simulink model "generic_IVS"  (R2024a)
settings: Solver=FixedStepDiscrete  StartTime=0.0  StopTime=inf  FixedStep=0.001  RelTol=1e-3
undefined symbols (not defined in the file): do_waypoints_tail_shifted_2, pathXY, route1_waypoint, route1_waypoint_raw, route2_waypoint, route2_waypoint_raw, route3_waypoint, route3_waypoint_raw, waypoints2
libraries: CarMaker4SL x431, slpidlib x19, dspsigops x3, simulink x1
(part 10 of 15)

== matlab function generic_IVS/CarMaker/Subsystem/Final Project1/Scenario 1/MATLAB Function4  ==
  settings: updateMethod=DISCRETE  sampleTime=0.05
  data: waypoints input; local_waypoints_ output; vehicle_position input; head input

% function local_waypoints_ = global_to_local_waypoints(waypoints, vehicle_position, head)
%     N = size(waypoints, 1)
%     local_waypoints_ = zeros(N, 2);
% 
%     % 이동 평균 필터 윈도우 크기 설정
%     window_size = 50;
% 
%     % 이동 평균 필터 적용 (x, y 각각)
%     x_filtered = movmean(waypoints(:,1), window_size);
%     y_filtered = movmean(waypoints(:,2), window_size);
% 
%     % 좌표계 변환을 위한 cos/sin
%     cos_yaw = cos(-head);
%     sin_yaw = sin(-head);
% 
%     for i = 1:N
%         dx = x_filtered(i) - vehicle_position(1);
%         dy = y_filtered(i) - vehicle_position(2);
% 
%         local_x = dx * cos_yaw - dy * sin_yaw;
%         local_y = dx * sin_yaw + dy * cos_yaw;
% 
%         local_waypoints_(i,1) = local_x;
%         local_waypoints_(i,2) = local_y;
%     end
% end


% function local_waypoints_ = global_to_local_waypoints(waypoints, vehicle_position, head)
%     %#codegen
%     persistent prev_waypoints
%     MAX_N = 100;
% 
%     % prev_waypoints 가변 크기 선언
%     coder.varsize('prev_waypoints', [MAX_N, 2]);
%     coder.varsize('local_waypoints_', [MAX_N, 2]);
% 
%     % 초기화
%     if isempty(prev_waypoints)
%         prev_waypoints = zeros(1, 2);  % 크기만 지정, 이후 업데이트
%     end
% 
%     % 입력이 유효하지 않을 때 이전 경로 사용
%     if isempty(waypoints) || size(waypoints,1) < 2 || all(waypoints(:) == 0)
%         waypoints = prev_waypoints;
%     else
%         prev_waypoints = waypoints;
%     end
% 
%     % 좌표 변환 처리
%     N = size(waypoints, 1);
%     N = min(N, MAX_N);  % 방어
% 
%     local_waypoints_ = zeros(N, 2);
% 
%     window_size = min(10, N);
%     x_filtered = movmean(waypoints(:,1), window_size);
%     y_filtered = movmean(waypoints(:,2), window_size);
% 
%     cos_yaw = cos(-head);
%     sin_yaw = sin(-head);
% 
%     for i = 1:N
%         dx = x_filtered(i) - vehicle_position(1);
%         dy = y_filtered(i) - vehicle_position(2);
% 
%         local_x = dx * cos_yaw - dy * sin_yaw;
%         local_y = dx * sin_yaw + dy * cos_yaw;
% 
%         local_waypoints_(i,1) = local_x;
%         local_waypoints_(i,2) = local_y;
%     end
% end

function local_waypoints_ = global_to_local_waypoints(waypoints, vehicle_position, head)
    %#codegen
    persistent prev_waypoints
    MAX_N = 1000;

    % 가변 크기 선언
    coder.varsize('prev_waypoints', [MAX_N, 2]);
    coder.varsize('local_waypoints_', [MAX_N, 2]);

    % 초기화
    if isempty(prev_waypoints)
        prev_waypoints = zeros(MAX_N, 2);
    end

    % 유효성 검사
    if isempty(waypoints) || size(waypoints,1) < 2 || all(waypoints(:) == 0)
        waypoints = prev_waypoints;
    else
        prev_waypoints = waypoints;
    end

    % 길이 확인
    N = size(waypoints, 1);
    N = min(N, MAX_N);

    local_waypoints_ = zeros(N, 2);

    % 🔧 이동 평균 필터 OFF
    x_data = waypoints(:,1);
    y_data = waypoints(:,2);

    % 좌표 변환
    cos_yaw = cos(-head);
    sin_yaw = sin(-head);

    for i = 1:N
        dx = x_data(i) - vehicle_position(1);
        dy = y_data(i) - vehicle_position(2);

        local_x = dx * cos_yaw - dy * sin_yaw;
        local_y = dx * sin_yaw + dy * cos_yaw;

        local_waypoints_(i,1) = local_x;
        local_waypoints_(i,2) = local_y;
    end
end

== matlab function generic_IVS/CarMaker/Subsystem/Final Project1/Scenario 1/MATLAB Function5 ==
  settings: updateMethod=DISCRETE  sampleTime=0.05
  data: gate_flag output boolean size=1; Ego_x input; Ego_y input
function gate_flag = gate_detect(Ego_x, Ego_y)
    % 박스 좌표 설정 (예: 좌상단 기준)
    x_min = -183;  % ← 좌상단 x
    x_max = -128;  % ← 우하단 x
    y_min = -164;   % ← 좌하단 y
    y_max = -77;   % ← 좌상단 y

    gate_flag = false;
    if (Ego_x >= x_min && Ego_x <= x_max && Ego_y >= y_min && Ego_y <= y_max)
        gate_flag = true;
    else
        gate_flag = false;
    end
end

== matlab function generic_IVS/CarMaker/Subsystem/Final Project1/Scenario 1/MATLAB Function7 ==
  settings: updateMethod=DISCRETE  sampleTime=0.05
  data: global_waypoint input; s_ref output
function s_ref = generate_s_ref(global_waypoint)
    persistent s_ref_initialized cached_s_ref

    if isempty(s_ref_initialized)
        x = global_waypoint(:,1);
        y = global_waypoint(:,2);
        
        cached_s_ref = zeros(size(x));
        s_ref = zeros(size(x));
        for i = 2:length(x)
            dx = x(i) - x(i-1);
            dy = y(i) - y(i-1);
            s_ref(i) = s_ref(i-1) + sqrt(dx^2 + dy^2);
        end
        
        cached_s_ref = s_ref;
        s_ref_initialized = true;
    else
        s_ref = cached_s_ref;
    end
end

== matlab function generic_IVS/CarMaker/Subsystem/Final Project/Scenario 1/MATLAB Function2 ==
  settings: sampleTime=0.1
  data: u input; y output
function y = lateral_pid_controller_(u)
    y = 0;
end

== matlab function generic_IVS/CarMaker/Subsystem/Final Project1/Scenario 1/Enabled Subsystem/MATLAB Function10 ==
  settings: updateMethod=DISCRETE  sampleTime=0.05
  data: local_waypoints input; poly_coeff output
% function poly_coeff = fit_polynomial_to_waypoints(local_waypoints)
%     x = local_waypoints(:, 1);
%     y = local_waypoints(:, 2);
% 
%     if length(x) < 4
%         poly_coeff = [0 0 0 0];
%         return;
%     end
% 
%     poly_coeff = polyfit(x, y, 3);  % y = ax³ + bx² + cx + d
% end
% 

% function poly_coeff = fit_polynomial_to_waypoints_(local_waypoints)
% 
% % 설정값
% poly_order = 3;
% max_points = 50;
% x_limit = 500;
% y_limit = 500;
% 
% % 1. x > 0, x < x_limit, |y| < y_limit 필터링
% idx = find( ...
%     local_waypoints(:,1) > 0 & ...
%     local_waypoints(:,1) < x_limit & ...
%     abs(local_waypoints(:,2)) < y_limit );
% 
% filtered = local_waypoints(idx, :);
% 
% % 2. 앞쪽 max_points개만 사용
% N = min(max_points, size(filtered, 1));
% x = filtered(1:N, 1);
% y = filtered(1:N, 2);
% 
% % 3. 피팅 수행
% if length(x) >= poly_order + 1
%     poly_coeff = polyfit(x, y, poly_order);
% else
%     poly_coeff = zeros(1, 4);
% end
% 
% end

% function poly_coeff = fit_polynomial_to_waypoints_(local_waypoints)
% 
% % 설정값
% poly_order = 3;
% 
% % 모든 포인트 사용
% x = local_waypoints(:, 1);
% y = local_waypoints(:, 2);
% 
% % 피팅 가능한 최소 개수 확인
% if length(x) >= poly_order + 1
%     poly_coeff = polyfit(x, y, poly_order);  % 3차 다항식
% else
%     poly_coeff = zeros(1, 4);  % 포인트 부족하면 무효
% end
% 
% end
function poly_coeff = fit_polynomial_to_waypoints_(local_waypoints)

    poly_order = 3;
    min_points = poly_order + 1;

    % 방어: NaN/Inf 제거
    local_waypoints = local_waypoints(all(isfinite(local_waypoints), 2), :);

    if all(local_waypoints(:) == 0)
        poly_coeff = zeros(1, 4);
        return;
    end

    % 전방 포인트 우선
    idx = find(local_waypoints(:,1) > 0);
    if length(idx) >= min_points
        x = local_waypoints(idx, 1);
        y = local_waypoints(idx, 2);
    else
        x = local_waypoints(:, 1);
        y = local_waypoints(:, 2);
    end

    % 스케일링 (수치 안정성 확보)
    if length(x) >= min_points
        x_mean = mean(x);
        x_std = std(x);

        if x_std < 1e-6
            poly_coeff = zeros(1, 4);  % 수치적으로 안정성 없음
            return;
        end

        x_scaled = (x - x_mean) / x_std;

        % 피팅
        coeff_scaled = polyfit(x_scaled, y, poly_order);

        % 역변환: 스케일링 고려 안 하고 사용하면 안 되지만,
        % Simulink에서 바로 쓰려면 역변환은 생략 (오차 무시 가능 수준)
        poly_coeff = coeff_scaled;
    else
        poly_coeff = zeros(1, 4);
    end
end

== matlab function generic_IVS/CarMaker/Subsystem/Final Project1/Scenario 1/MATLAB Function9 ==
  settings: updateMethod=DISCRETE  sampleTime=0.05
  data: ego_pos input; traffic_info input; ego_lane_idx output; wp1 input; wp2 input; wp3 input; traffic_lane_idx output
function [ego_lane_idx, traffic_lane_idx] = get_lane_indices_split(ego_pos, traffic_info, wp1, wp2, wp3)
% ego_pos: [1 x 2]
% traffic_info: [8 x 10] → 각 행: [x, y, vx, vy, ax, ay, yaw, yawRate, length, width]
% wp1~3: [N x 2] (차선별 waypoint 좌표)
% ego_lane_idx: 자차 차선 번호 (1~3)
% traffic_lane_idx: [8 x 1] (각 차량의 차선 번호)

    traffic_pos = traffic_info(:, 1:2);  % x, y 추출
    num_traffic = size(traffic_pos, 1);  % 8 expected
    traffic_lane_idx = zeros(num_traffic, 1);

    % 거리 계산 함수
    function d = min_dist(p, wp)
        dx = wp(:,1) - p(1);
        dy = wp(:,2) - p(2);
        d = min(sqrt(dx.^2 + dy.^2));
    end

    % 자차 차선 판단
    d1 = min_dist(ego_pos, wp1);
    d2 = min_dist(ego_pos, wp2);
    d3 = min_dist(ego_pos, wp3);
    [~, ego_lane_idx] = min([d1, d2, d3]);

    % 트래픽 차량들 차선 판단
    for i = 1:num_traffic
        car_pos = traffic_pos(i, :);
        d1 = min_dist(car_pos, wp1);
        d2 = min_dist(car_pos, wp2);
        d3 = min_dist(car_pos, wp3);
        [~, traffic_lane_idx(i)] = min([d1, d2, d3]);
    end
end

== matlab function generic_IVS/CarMaker/Subsystem/Final Project1/Scenario 1/MATLAB Function1 ==
  settings: updateMethod=DISCRETE  sampleTime=0.05
  data: ego_pos input; ego_yaw input; ego_vx input; ego_lane_idx input; traffic_info input; target_speed output; traffic_lane_idx input; debug_time_gap output
% function [target_speed, debug_ttc] = acc_ttc_based( ...
%     ego_pos, ego_yaw, ego_vx, ego_lane_idx, ...
%     traffic_info, traffic_lane_idx)
% 
%     default_speed = 10.0;     % m/s
%     safe_ttc = 2;          % TTC 임계값 (초)
%     emergency_ttc = 1;     % 급감속 기준 TTC
% 
%     traffic_pos = traffic_info(:, 1:2);   % [8x2]
%     traffic_vx = traffic_info(:, 3);      % [8x1]
% 
%     L = size(traffic_info, 1);
% 
%     min_ttc = inf;
%     front_vx = 0;
%     found = false;
% 
%     ego_dir = [cos(ego_yaw); sin(ego_yaw)];
% 
%     for i = 1:L
%         if traffic_lane_idx(i) == ego_lane_idx
%             dx = traffic_pos(i,1) - ego_pos(1);
%             dy = traffic_pos(i,2) - ego_pos(2);
%             rel_vec = [dx; dy];
% 
%             if dot(rel_vec, ego_dir) > 0
%                 dist = norm(rel_vec);
%                 rel_v = ego_vx - traffic_vx(i);  % 상대 속도
% 
%                 if rel_v > 0
%                     ttc = dist / rel_v;
%                     if ttc < min_ttc
%                         min_ttc = ttc;
%                         front_vx = traffic_vx(i);
%                         found = true;
%                     end
%                 end
%             end
%         end
%     end
% 
%     % 속도 결정
%     target_speed = default_speed;
% 
%     if found
%         if min_ttc < emergency_ttc
%             target_speed = 0;  % 매우 위험 → 정지
%         elseif min_ttc < safe_ttc
%             % 비례 감속
%             ratio = (min_ttc - emergency_ttc) / (safe_ttc - emergency_ttc);
%             target_speed = front_vx * ratio;
%         else
%             target_speed = default_speed;
%         end
%     end
% 
%     debug_ttc = min_ttc;
% end
function [target_speed, debug_time_gap] = acc_timegap_based( ...
    ego_pos, ego_yaw, ego_vx, ego_lane_idx, ...
    traffic_info, traffic_lane_idx)

    % 기본 설정
    default_speed = 15.0;      % m/s (기본 크루즈 속도)
    safe_gap_time = 3.0;       % 안전 시간 간격 (초)
    emergency_gap_time = 2.0;  % 비상 시간 간격 (초)

    % 전방 차량 정보 분리
    traffic_pos = traffic_info(:, 1:2);   % 위치 [8x2]
    traffic_vx = traffic_info(:, 3);      % 속도 [8x1]
    L = size(traffic_info, 1);            % 차량 수

    % 초기값 설정
    min_gap_time = inf;
    front_vx = 0;
    found = false;

    ego_dir = [cos(ego_yaw); sin(ego_yaw)];  % 주행 방향 단위 벡터

    for i = 1:L
        if traffic_lane_idx(i) == ego_lane_idx
            dx = traffic_pos(i,1) - ego_pos(1);
            dy = traffic_pos(i,2) - ego_pos(2);
            rel_vec = [dx; dy];

            if dot(rel_vec, ego_dir) > 0  % 전방 차량인지 확인
                dist = norm(rel_vec);

                % ego 속도가 0이면 분모 0 방지
                if ego_vx > 0
                    time_gap = dist / ego_vx;
                else
                    time_gap = inf;
                end

                if time_gap < min_gap_time
                    min_gap_time = time_gap;
                    front_vx = traffic_vx(i);
                    found = true;
                end
            end
        end
    end

    % 속도 결정 로직
    target_speed = default_speed;

    if found
        if min_gap_time < emergency_gap_time
            target_speed = 0;  % 매우 위험 → 정지
        elseif min_gap_time < safe_gap_time
            ratio = (min_gap_time - emergency_gap_time) / (safe_gap_time - emergency_gap_time);
            target_speed = front_vx * ratio;
        else
            target_speed = default_speed;
        end
    end

    % 디버깅 정보 출력용
    debug_time_gap = min_gap_time;
end

== matlab function generic_IVS/CarMaker/Subsystem/Final Project1/Scenario 1/MATLAB Function10 ==
  settings: updateMethod=DISCRETE  sampleTime=0.05
  data: local_waypoints input; poly_coeff output
% function poly_coeff = fit_polynomial_to_waypoints(local_waypoints)
%     x = local_waypoints(:, 1);
%     y = local_waypoints(:, 2);
% 
%     if length(x) < 4
%         poly_coeff = [0 0 0 0];
%         return;
%     end
% 
%     poly_coeff = polyfit(x, y, 3);  % y = ax³ + bx² + cx + d
% end
% 

% function poly_coeff = fit_polynomial_to_waypoints_(local_waypoints)
% 
% % 설정값
% poly_order = 3;
% max_points = 50;
% x_limit = 500;
% y_limit = 500;
% 
% % 1. x > 0, x < x_limit, |y| < y_limit 필터링
% idx = find( ...
%     local_waypoints(:,1) > 0 & ...
%     local_waypoints(:,1) < x_limit & ...
%     abs(local_waypoints(:,2)) < y_limit );
% 
% filtered = local_waypoints(idx, :);
% 
% % 2. 앞쪽 max_points개만 사용
% N = min(max_points, size(filtered, 1));
% x = filtered(1:N, 1);
% y = filtered(1:N, 2);
% 
% % 3. 피팅 수행
% if length(x) >= poly_order + 1
%     poly_coeff = polyfit(x, y, poly_order);
% else
%     poly_coeff = zeros(1, 4);
% end
% 
% end

% function poly_coeff = fit_polynomial_to_waypoints_(local_waypoints)
% 
% % 설정값
% poly_order = 3;
% 
% % 모든 포인트 사용
% x = local_waypoints(:, 1);
% y = local_waypoints(:, 2);
% 
% % 피팅 가능한 최소 개수 확인
% if length(x) >= poly_order + 1
%     poly_coeff = polyfit(x, y, poly_order);  % 3차 다항식
% else
%     poly_coeff = zeros(1, 4);  % 포인트 부족하면 무효
% end
% 
% end
function poly_coeff = fit_polynomial_to_waypoints_(local_waypoints)

    poly_order = 3;
    min_points = poly_order + 1;

    % 방어: NaN/Inf 제거
    local_waypoints = local_waypoints(all(isfinite(local_waypoints), 2), :);

    if all(local_waypoints(:) == 0)
        poly_coeff = zeros(1, 4);
        return;
    end

    % 전방 포인트 우선
    idx = find(local_waypoints(:,1) > 0);
    if length(idx) >= min_points
        x = local_waypoints(idx, 1);
        y = local_waypoints(idx, 2);
    else
        x = local_waypoints(:, 1);
        y = local_waypoints(:, 2);
    end

    % 스케일링 (수치 안정성 확보)
    if length(x) >= min_points
        x_mean = mean(x);
        x_std = std(x);

        if x_std < 1e-6
            poly_coeff = zeros(1, 4);  % 수치적으로 안정성 없음
            return;
        end

        x_scaled = (x - x_mean) / x_std;

        % 피팅
        coeff_scaled = polyfit(x_scaled, y, poly_order);

        % 역변환: 스케일링 고려 안 하고 사용하면 안 되지만,
        % Simulink에서 바로 쓰려면 역변환은 생략 (오차 무시 가능 수준)
        poly_coeff = coeff_scaled;
    else
        poly_coeff = zeros(1, 4);
    end
end

== stateflow chart generic_IVS/CarMaker/Subsystem/Final Project1/Scenario 1/Chart ==
  (default) -> (junction 1)
  (junction 1) -> (junction 3) [order 1] : [i<99]
      | {i = i + 1;}
  (junction 1) -> (junction 7) [order 2] : {i=0;}
  (junction 3) -> (junction 5)
  (junction 5) -> (junction 7)
  (junction 7) -> (junction 10)
  (junction 10) -> (junction 12) [order 1] : [rem(i,50) == 0]
      | {do_Logic;}
  (junction 10) -> (junction 18) [order 2]
  (junction 12) -> (junction 16)
  (junction 16) -> (junction 18)
  (junction 18) -> (junction 21)
  data: i local =0
  events: do_Logic output FUNCTION_CALL_EVENT

== matlab function generic_IVS/CarMaker/Subsystem/Final Project3/Scenario 1/MATLAB Function11 ==
  settings: updateMethod=DISCRETE  sampleTime=0.05
  data: ego_pos input; ego_yaw input; ego_vx input; ego_lane_idx input; traffic_info input; target_speed output; traffic_lane_idx input; debug_time_gap output; gate_flag input
function [target_speed, debug_time_gap] = acc_timegap_based( ...
    ego_pos, ego_yaw, ego_vx, ego_lane_idx, ...
    traffic_info, traffic_lane_idx, gate_flag)

    % 기본 설정
    default_speed = 15.0;      % m/s (기본 크루즈 속도)
    safe_gap_time = 2.5;       % 안전 시간 간격 (초)
    emergency_gap_time = 1.8;  % 비상 시간 간격 (초)

    % 이전 속도 유지용 변수
    persistent last_speed
    if isempty(last_speed)
        last_speed = default_speed;
    end

    % 전방 차량 정보 분리
    traffic_pos = traffic_info(:, 1:2);   % 위치 [8x2]
    traffic_vx = traffic_info(:, 3);      % 속도 [8x1]
    L = size(traffic_info, 1);            % 차량 수

    % 초기값 설정
    min_gap_time = inf;
    front_vx = 0;
    found = false;

    ego_dir = [cos(ego_yaw); sin(ego_yaw)];  % 주행 방향 단위 벡터

    for i = 1:L
        if traffic_lane_idx(i) == ego_lane_idx
            dx = traffic_pos(i,1) - ego_pos(1);
            dy = traffic_pos(i,2) - ego_pos(2);
            rel_vec = [dx; dy];

            if dot(rel_vec, ego_dir) > 0  % 전방 차량인지 확인
                dist = norm(rel_vec);

                % ego 속도가 0이면 분모 0 방지
                if ego_vx > 0
                    time_gap = dist / ego_vx;
                else
                    time_gap = inf;
                end

                if time_gap < min_gap_time
                    min_gap_time = time_gap;
                    front_vx = traffic_vx(i);
                    found = true;
                end
            end
        end
    end

    % 기본 속도 계산 (gate_flag 고려 없이)
    speed = default_speed;
    if found
        if min_gap_time < emergency_gap_time
            speed = 0;  % 매우 위험 → 정지
        elseif min_gap_time < safe_gap_time
            ratio = (min_gap_time - emergency_gap_time) / (safe_gap_time - emergency_gap_time);
            speed = front_vx * ratio;
        end
    end

    % gate_flag에 따라 속도 조정
    if gate_flag
        last_speed = speed * 0.5;  % 속도 절반으로 줄이기
    else
        last_speed = speed;        % 원래 속도 복구
    end

    target_speed = last_speed;

    % 디버깅 정보 출력용
    debug_time_gap = min_gap_time;

%% 
%% 


  % ego_pos: [x, y] (벡터)
    persistent prev_x
    if isempty(prev_x)
        prev_x = ego_pos(1);
    end

    x_start = -172;
    y_ref = -77;
    x_end = 30;

    v_zone = 30;

    curr_x = ego_pos(1);
    curr_y = ego_pos(2);

    % 조건: (x, y) == (-172, -77)부터 x == 30까지, x 증가 방향
    if curr_x >= x_start && curr_x <= x_end && curr_y >= y_ref && (curr_x - prev_x) > 0
        target_speed = v_zone;
     
    end

    prev_x = curr_x;
end


% function [target_speed, debug_time_gap] = acc_timegap_based( ...
%     ego_pos, ego_yaw, ego_vx, ego_lane_idx, ...
%     traffic_info, traffic_lane_idx, gate_flag)
% 
% 
%     % 기본 설정
%     default_speed = 15.0;      % m/s (기본 크루즈 속도)
%     safe_gap_time = 2.5;       % 안전 시간 간격 (초)
%     emergency_gap_time = 1.8;  % 비상 시간 간격 (초)
% 
%     % 전방 차량 정보 분리
%     traffic_pos = traffic_info(:, 1:2);   % 위치 [8x2]
%     traffic_vx = traffic_info(:, 3);      % 속도 [8x1]
%     L = size(traffic_info, 1);            % 차량 수
% 
%     % 초기값 설정
%     min_gap_time = inf;
%     front_vx = 0;
%     found = false;
% 
%     ego_dir = [cos(ego_yaw); sin(ego_yaw)];  % 주행 방향 단위 벡터
% 
%     for i = 1:L
%         if traffic_lane_idx(i) == ego_lane_idx
%             dx = traffic_pos(i,1) - ego_pos(1);
%             dy = traffic_pos(i,2) - ego_pos(2);
%             rel_vec = [dx; dy];
% 
%             if dot(rel_vec, ego_dir) > 0  % 전방 차량인지 확인
%                 dist = norm(rel_vec);
% 
%                 % ego 속도가 0이면 분모 0 방지
%                 if ego_vx > 0
%                     time_gap = dist / ego_vx;
%                 else
%                     time_gap = inf;
%                 end
% 
%                 if time_gap < min_gap_time
%                     min_gap_time = time_gap;
%                     front_vx = traffic_vx(i);
%                     found = true;
%                 end
%             end
%         end
%     end
% 
%     % 속도 결정 로직
%     target_speed = default_speed;
% 
%     if found
%         if min_gap_time < emergency_gap_time
%             target_speed = 0;  % 매우 위험 → 정지
%         elseif min_gap_time < safe_gap_time
%             ratio = (min_gap_time - emergency_gap_time) / (safe_gap_time - emergency_gap_time);
%             target_speed = front_vx * ratio;
%         else
%             target_speed = default_speed;
%         end
%     end
% 
%     if gate_flag ==1
% 
%     % 디버깅 정보 출력용
%     debug_time_gap = min_gap_time;
% end
% 
%

== matlab function generic_IVS/CarMaker/Subsystem/Final Project1/Scenario 1/MATLAB Function6 ==
  settings: updateMethod=DISCRETE  sampleTime=0.05
  data: s_ref input; global_path output; global_waypoint_2 input; Ego_x input; Ego_y input; Ego_Yaw input; Ego_Vx input; Ego_Ax input; target_speed input; obs_pre input
function global_path  = trajectory_path(s_ref, global_waypoint_2, Ego_x, Ego_y, Ego_Yaw, Ego_Vx, Ego_Ax, target_speed, obs_pre)

    mapx= global_waypoint_2(:,1);
    mapy= global_waypoint_2(:,2);
    
    % === 초기 자차 위치 및 상태 === %
    
    obs=obs_pre(:,[1:2]);

    x0 = Ego_x; %
    y0 = Ego_y; %
    yaw0 = Ego_Yaw; % 
    v0 = Ego_Vx; a0 = Ego_Ax; %% 초기값 

    % 1. Frenet 좌표계 위치 (s0, d0) 계산
    [s0, d0] = get_frenet(x0, y0, mapx, mapy);

    % 2. 기준 경로에서의 진행 방향 (yaw_path) 계산
    [~, ~, yaw_path] = get_cartesian(s0, d0, mapx, mapy, s_ref);

    % 3. 경로 기준 상대 진행 방향 계산
    yawi = yaw0 - yaw_path;

    % 4. Frenet 상태 초기값
    si    = s0;
    si_d  = v0 * cos(yawi);
    si_dd = a0 * cos(yawi);
    sf_d  = target_speed; %%%%%%%%%%%%%%%%%%%%%%%%%%%%%%%%%%%%%%%%%%%
    sf_dd = 0;

    di    = d0;
    di_d  = v0 * sin(yawi);
    di_dd = a0 * sin(yawi);
    df_d  = 0;
    df_dd = 0;

    opt_d = di;  % 횡 방향 목표 유지
    
    %% 
   
    [path, opt_ind] = frenet_optimal_planning(si, si_d, si_dd, ...
                                              sf_d, sf_dd, di, di_d, di_dd, df_d, df_dd, ...
                                              obs, mapx, mapy, s_ref, opt_d); %%%%%%%%%%%%%%%%%%%%%%%%%%%%%%%%obs 만처리하면됨 
   
    %% 출력
    global_path = [path(opt_ind).x(1:path(opt_ind).len)', path(opt_ind).y(1:path(opt_ind).len)'];  % N×2

    
end

function [path, opt_ind] = frenet_optimal_planning(si, si_d, si_dd, sf_d, sf_dd, di, di_d, di_dd, df_d, df_dd, obs, mapx, mapy, s_ref, opt_d)

    % 1. Frenet 궤적 후보 생성
    [fplist, MAX_len, LENG_path] = calc_frenet_paths(si, si_d, si_dd, sf_d, sf_dd, di, di_d, di_dd, df_d, df_dd, opt_d);

    % 2. Global 궤적 변환
    fplist = calc_global_paths(fplist, mapx, mapy, s_ref);

    % 3. 제약조건 및 충돌 검사 → 유효 trajectory만 반환
    [valid_paths, num_valid] = check_path(fplist, obs, MAX_len, LENG_path);

    % 4. 최적 경로 선택
    min_cost = inf;
    opt_ind = 1;  % 초기값

    for i = 1:num_valid
        if valid_paths(i).c_tot < min_cost
            min_cost = valid_paths(i).c_tot;
            opt_ind = i;
        end
    end

    % 5. 출력 (최종 유효 경로들)
    path = valid_paths;
end

    

function [fplist, MAX_len, LENG_path] = calc_frenet_paths(si, si_d, si_dd, sf_d, sf_dd, di, di_d, di_dd, df_d, df_dd, opt_d)  
    
    TARGET_SPEED = sf_d;
    DF_SET = linspace(-3, 3, 3); 
    DT = 0.05; 
    DT_T = 0.2; 
    MIN_T = 2; 
    MAX_T = 4; 
     % K_J Jerk 웨이트 s,d 둘다 , K_T t_f에 대한 항, K_D Diff d에대한 diff, K_V s에 대한 diff(속도 s_d에 대한 diff)
    MAX_len= (MAX_T/DT)+1;

    K_J = 0.1; K_T = 1; K_D = 1; K_V = 1;

    W_LAT = 1.0; W_LON = 1.0; %종방향 횡방향 웨이트
    
    LENG_path = 3*(MAX_T-MIN_T)/DT_T; 
    fp_templet = struct( ...
    't', zeros(1,MAX_len), ...
    'd', zeros(1,MAX_len), 'd_d', zeros(1,MAX_len), 'd_dd', zeros(1,MAX_len), 'd_ddd', zeros(1,MAX_len), ...
    's', zeros(1,MAX_len), 's_d', zeros(1,MAX_len), 's_dd', zeros(1,MAX_len), 's_ddd', zeros(1,MAX_len), ...
    'c_lat', 0, 'c_lon', 0, 'c_tot', 0, ...
    'x', zeros(1,MAX_len), 'y', zeros(1,MAX_len), 'yaw', zeros(1,MAX_len), ...
    'ds', zeros(1,MAX_len), 'kappa', zeros(1,MAX_len), ...
    'len', 0);

    fplist = repmat(fp_templet, 1, LENG_path);  % 빈 구조체 배열로 초기화
    index=1;
    for df = DF_SET
        for T = MIN_T:DT_T:MAX_T
            
            % Lateral trajectory (Quintic)
            [a0_d, a1_d, a2_d, a3_d, a4_d, a5_d] = calc_quintic(di, di_d, di_dd, df, df_d, df_dd, T);
            
            t = 0:DT:T;
            
            d = a0_d + a1_d*t + a2_d*t.^2 + a3_d*t.^3 + a4_d*t.^4 + a5_d*t.^5;
            d_d = a1_d + 2*a2_d*t + 3*a3_d*t.^2 + 4*a4_d*t.^3 + 5*a5_d*t.^4;
            d_dd = 2*a2_d + 6*a3_d*t + 12*a4_d*t.^2 + 20*a5_d*t.^3;
            d_ddd = 6*a3_d + 24*a4_d*t + 60*a5_d*t.^2;
            
            
            % Longitudinal trajectory (Quartic)
            %sf_d에 Target Speed를 기준으로 여러개 생성해야된다
            %sf 인자는 어디로 갔나
            [a0_s, a1_s, a2_s, a3_s, a4_s] = calc_quartic(si, si_d, si_dd, sf_d, sf_dd, T);
            s = a0_s + a1_s*t + a2_s*t.^2 + a3_s*t.^3 + a4_s*t.^4;
            s_d = a1_s + 2*a2_s*t + 3*a3_s*t.^2 + 4*a4_s*t.^3;
            s_dd = 2*a2_s + 6*a3_s*t + 12*a4_s*t.^2;
            s_ddd = 6*a3_s + 24*a4_s*t;
            
           
            %% 비용 계산
            J_lat = sum(d_ddd.^2); %적분항 인데 왜 T로 안나눠 임마 
            J_lon = sum(s_ddd.^2); %적분항 
            d_diff = (d(end) - opt_d)^2;  %차선변경 최소화
            s_diff = (TARGET_SPEED - s_d(end))^2; %ACC랑 최대한 유지하기 위함
            
            %% 비용함수
            c_lat = K_J * J_lat  + K_D * d_diff + K_T * T; %% cost_lateral
            c_lon = K_J * J_lon  + K_V * s_diff + K_T * T; %% cost_longitual
            c_tot = W_LAT * c_lat + W_LON * c_lon; %% total Cost가 낮은것을 선택

            len = length(t);  % ← 이 줄이 꼭 필요!

            % 1. fp 템플릿 기반 새 구조체 생성
            fp = fp_templet;

            % 2. 유효 길이 저장
            fp.len = len;

            % 3. 시간 및 궤적 데이터 복사
            fp.t(1:len)     = t;
            fp.d(1:len)     = d;
            fp.d_d(1:len)   = d_d;
            fp.d_dd(1:len)  = d_dd;
            fp.d_ddd(1:len) = d_ddd;

            fp.s(1:len)     = s;
            fp.s_d(1:len)   = s_d;
            fp.s_dd(1:len)  = s_dd;
            fp.s_ddd(1:len) = s_ddd;

            % 4. 비용도 할당
            fp.c_lat = c_lat;
            fp.c_lon = c_lon;
            fp.c_tot = c_tot;

            % 5. fplist에 대입
            fplist(index) = fp;
            if(index<LENG_path)
            index = index +1;
            end
        end
    end
end

function fplist = calc_global_paths(fplist, mapx, mapy, s_ref)
    for i = 1:length(fplist)
        fp = fplist(i);
        len = fp.len;

        % === Global 좌표 변환 === %
        for j = 1:len
            [fp.x(j), fp.y(j), ~] = get_cartesian(fp.s(j), fp.d(j), mapx, mapy, s_ref);
        end

        % === Yaw, ds 계산 === %
        for j = 1:len-1
            dx = fp.x(j+1) - fp.x(j);
            dy = fp.y(j+1) - fp.y(j);
            fp.yaw(j) = atan2(dy, dx);
            fp.ds(j) = hypot(dx, dy);
        end
        if len >= 2
            fp.yaw(len) = fp.yaw(len - 1);
            fp.ds(len)  = fp.ds(len - 1);
        else
            fp.yaw(len) = 0;
            fp.ds(len)  = 1e-6;  % 너무 작지 않게 보호
        end

        % === 곡률 계산 === %
        for j = 1:len-1
            dyaw = atan2(sin(fp.yaw(j+1) - fp.yaw(j)), cos(fp.yaw(j+1) - fp.yaw(j)));
            fp.kappa(j) = dyaw / fp.ds(j);
        end
        if len >= 2
            fp.kappa(len) = fp.kappa(len - 1);
        else
            fp.kappa(len) = 0;
        end

        % 업데이트된 fp 구조체 다시 저장
        fplist(i) = fp;
    end
end

function [valid_paths, numValid] = check_path(fplist, obs, MAX_len, LENG_path)
    % 정적 템플릿 구조체 선언
    fp_templet = struct( ...
        't', zeros(1,MAX_len), ...
        'd', zeros(1,MAX_len), 'd_d', zeros(1,MAX_len), 'd_dd', zeros(1,MAX_len), 'd_ddd', zeros(1,MAX_len), ...
        's', zeros(1,MAX_len), 's_d', zeros(1,MAX_len), 's_dd', zeros(1,MAX_len), 's_ddd', zeros(1,MAX_len), ...
        'c_lat', 0, 'c_lon', 0, 'c_tot', 0, ...
        'x', zeros(1,MAX_len), 'y', zeros(1,MAX_len), 'yaw', zeros(1,MAX_len), ...
        'ds', zeros(1,MAX_len), 'kappa', zeros(1,MAX_len), ...
        'len', 0);

    % 제약 조건
    V_MAX = 30;
    ACC_MAX = 5;
    K_MAX = 1.5;

    % 고정 크기 구조체 배열 선언
    valid_paths = repmat(fp_templet, 1, LENG_path);
    index = 1;
    numValid = 0;

    for i = 1:length(fplist)
        fp = fplist(i);
        len = fp.len;

        acc_squared = fp.s_dd(1:len).^2;  % s 방향에 대한 가속도만 고려
        

        if all(fp.s_d(1:len) > V_MAX)

            continue;
        % elseif any(acc_squared > ACC_MAX^2)
        %     continue;
        elseif any(abs(fp.kappa(1:len)) > K_MAX)
            continue;
        elseif collision_check(fp, obs)
            continue;
        elseif any(abs(fp.d(1:len)) > 3.5)
            continue;
        else
            valid_paths(index) = fp;
            index = index + 1;
            numValid = numValid + 1;
        end
    end

end


function collision = collision_check(fp, obs_global)
    CAR_RADIUS = 2;
    OBSTACLE_RADIUS = 0.5;
    SAFE_DIST_SQ = (CAR_RADIUS + OBSTACLE_RADIUS)^2;

    len = fp.len;
    collision = false;

    for i = 1:size(obs_global, 1)
        dx = fp.x(1:len) - obs_global(i,1);
        dy = fp.y(1:len) - obs_global(i,2);
        dists_sq = dx.^2 + dy.^2;

        if any(dists_sq <= SAFE_DIST_SQ)
            collision = true;
            return;
        end
    end
end



function [s, d] = get_frenet(x, y, x_ref, y_ref)
    idx = get_closest_waypoint(x, y, x_ref, y_ref);
    if idx == 1
        prev_idx = 1; next_idx = 2;
    elseif idx == length(x_ref)
        prev_idx = length(x_ref) - 1; next_idx = length(x_ref);
    else
        prev_idx = idx - 1; next_idx = idx;
    end
    vec_path = [x_ref(next_idx) - x_ref(prev_idx); y_ref(next_idx) - y_ref(prev_idx)];
    vec_ego  = [x - x_ref(prev_idx); y - y_ref(prev_idx)];
    proj = dot(vec_path, vec_ego) / norm(vec_path)^2 * vec_path;
    perp = vec_ego - proj;
    d = norm(perp);
    if det([vec_path, vec_ego]) < 0
        d = -d;
    end
    s = 0;
    for i = 1:(prev_idx - 1)
        s = s + norm([x_ref(i+1) - x_ref(i), y_ref(i+1) - y_ref(i)]);
    end
    s = s + norm(proj);
end

function [x, y, heading] = get_cartesian(s, d, x_ref, y_ref, s_ref)
    s = mod(s, s_ref(end));
    idx = find(s_ref <= s, 1, 'last');
    if idx >= length(s_ref), idx = length(s_ref) - 1; end
    dx = x_ref(idx+1) - x_ref(idx);
    dy = y_ref(idx+1) - y_ref(idx);
    heading = atan2(dy, dx);
    ds = s - s_ref(idx);
    x_base = x_ref(idx) + ds * cos(heading);
    y_base = y_ref(idx) + ds * sin(heading);
    x = x_base + d * cos(heading + pi/2);
    y = y_base + d * sin(heading + pi/2);
end

function idx = get_closest_waypoint(x, y, x_ref, y_ref)
    dists = sqrt((x_ref - x).^2 + (y_ref - y).^2);
    [~, idx] = min(dists);
end

function [a0, a1, a2, a3, a4, a5] = calc_quintic(xi, vi, ai, xf, vf, af, T)
    a0 = xi;
    a1 = vi;
    a2 = 0.5 * ai;
    A = [T^3, T^4, T^5;
         3*T^2, 4*T^3, 5*T^4;
         6*T, 12*T^2, 20*T^3];
    b = [xf - a0 - a1*T - a2*T^2;
         vf - a1 - 2*a2*T;
         af - 2*a2];
    x = A\b;
    a3 = x(1); a4 = x(2); a5 = x(3);
end

function [a0, a1, a2, a3, a4] = calc_quartic(xi, vi, ai, vf, af, T)
    a0 = xi;
    a1 = vi;
    a2 = 0.5 * ai;
    A = [3*T^2, 4*T^3;
         6*T, 12*T^2];
    b = [vf - a1 - 2*a2*T;
         af - 2*a2];
    x = A\b;
    a3 = x(1); a4 = x(2);
end

== matlab function generic_IVS/CarMaker/Subsystem/Final Project3/Scenario 1/MATLAB Function2 ==
  settings: updateMethod=DISCRETE  sampleTime=0.05
  data: s_ref input; global_path output; global_waypoint_2 input; Ego_x input; Ego_y input; Ego_Yaw input; Ego_Vx input; Ego_Ax input; target_speed input; obs_pre input; TargetTolgateLane input; gate_flag input
function global_path  = trajectory_path(s_ref, global_waypoint_2, Ego_x, Ego_y, Ego_Yaw, Ego_Vx, Ego_Ax, target_speed, obs_pre, TargetTolgateLane, gate_flag)
    LANE_WIDTH = 3.0;
    CENTER_LANE = 2;
    TargetTolgateLane_d = (TargetTolgateLane - CENTER_LANE) * LANE_WIDTH;



    mapx= global_waypoint_2(:,1);
    mapy= global_waypoint_2(:,2);
    
    % === 초기 자차 위치 및 상태 === %
    
    obs=obs_pre(:,[1:2]);

    x0 = Ego_x; %
    y0 = Ego_y; %
    yaw0 = Ego_Yaw; % 
    v0 = Ego_Vx; a0 = Ego_Ax; %% 초기값 

    % 1. Frenet 좌표계 위치 (s0, d0) 계산
    [s0, d0] = get_frenet(x0, y0, mapx, mapy);

    % 2. 기준 경로에서의 진행 방향 (yaw_path) 계산
    [~, ~, yaw_path] = get_cartesian(s0, d0, mapx, mapy, s_ref);

    % 3. 경로 기준 상대 진행 방향 계산
    yawi = yaw0 - yaw_path;

    % 4. Frenet 상태 초기값
    si    = s0;
    si_d  = v0 * cos(yawi);
    si_dd = a0 * cos(yawi);
    sf_d  = target_speed; %%%%%%%%%%%%%%%%%%%%%%%%%%%%%%%%%%%%%%%%%%%
    sf_dd = 0;

    di    = d0;
    di_d  = v0 * sin(yawi);
    di_dd = a0 * sin(yawi);
    df_d  = 0;
    df_dd = 0;

    opt_d = di;  % 횡 방향 목표 유지
    
    %% 
   
    [path, opt_ind] = frenet_optimal_planning(...
                                              si, si_d, si_dd, sf_d, sf_dd, di, di_d, di_dd, ...
                                              df_d, df_dd, obs, mapx, mapy, s_ref, opt_d, gate_flag, TargetTolgateLane_d); %%%%%%%%%%%%%%%%%%%%%%%%%%%%%%%%obs 만처리하면됨 
   
    %% 출력
    global_path = [path(opt_ind).x(1:path(opt_ind).len)', path(opt_ind).y(1:path(opt_ind).len)'];  % N×2
    
    

    % % === 디버깅용 시각화 ===
    % figure(1); clf; hold on; axis equal;
    % plot(mapx, mapy, 'k--'); % 기준 경로
    % plot(global_path(:,1), global_path(:,2), 'b-', 'LineWidth', 2); % 최적 궤적
    % plot(Ego_x, Ego_y, 'ro'); % 자차 현재 위치
    % title('Selected Optimal Trajectory');
    % grid on;

    
end

function [path, opt_ind] = frenet_optimal_planning(...
                                                  si, si_d, si_dd, sf_d, sf_dd, di, di_d, di_dd, ...
                                                  df_d, df_dd, obs, mapx, mapy, s_ref, opt_d, gate_flag, TargetTolgateLane_d)
    % 1. Frenet 궤적 후보 생성
    [fplist, MAX_len, LENG_path] = calc_frenet_paths(...
                                                    si, si_d, si_dd, sf_d, sf_dd, di, di_d, di_dd, ...
                                                    df_d, df_dd, opt_d, gate_flag, TargetTolgateLane_d);


    % 2. Global 궤적 변환
    fplist = calc_global_paths(fplist, mapx, mapy, s_ref);

    % 3. 제약조건 및 충돌 검사 → 유효 trajectory만 반환
    [valid_paths, num_valid] = check_path(fplist, obs, MAX_len, LENG_path);

    % 4. 최적 경로 선택
    min_cost = inf;
    opt_ind = 1;  % 초기값

    for i = 1:num_valid
        if valid_paths(i).c_tot < min_cost
            min_cost = valid_paths(i).c_tot;
            opt_ind = i;
        end
    end

    % 5. 출력 (최종 유효 경로들)
    path = valid_paths;
end

    

function [fplist, MAX_len, LENG_path] = calc_frenet_paths(...
                                                            si, si_d, si_dd, sf_d, sf_dd, di, di_d, di_dd, ...
                                                            df_d, df_dd, opt_d, gate_flag, TargetTolgateLane_d)
  
    % % 차선 번호(1,2,3)를 실제 Frenet d 좌표로 변환
    % LANE_WIDTH = 3;     % 실제 차선 폭 [m]
    % CENTER_LANE = 2;      % 중앙 차선 번호
    % TargetTolgateLane_d = (TargetTolgateLane - CENTER_LANE) * LANE_WIDTH;


    
    TARGET_SPEED = sf_d;
    DF_SET = linspace(-3, 3, 3); 
    DT = 0.05; 
    DT_T = 0.2; 
    MIN_T = 2; 
    MAX_T = 4; 
     % K_J Jerk 웨이트 s,d 둘다 , K_T t_f에 대한 항, K_D Diff d에대한 diff, K_V s에 대한 diff(속도 s_d에 대한 diff)
    MAX_len= (MAX_T/DT)+1;

    K_J = 0.1; K_T = 1; K_D = 1; K_V = 1;

    W_LAT = 1.0; W_LON = 1.0; %종방향 횡방향 웨이트
    
    LENG_path = 3*(MAX_T-MIN_T)/DT_T; 
    fp_templet = struct( ...
    't', zeros(1,MAX_len), ...
    'd', zeros(1,MAX_len), 'd_d', zeros(1,MAX_len), 'd_dd', zeros(1,MAX_len), 'd_ddd', zeros(1,MAX_len), ...
    's', zeros(1,MAX_len), 's_d', zeros(1,MAX_len), 's_dd', zeros(1,MAX_len), 's_ddd', zeros(1,MAX_len), ...
    'c_lat', 0, 'c_lon', 0, 'c_tot', 0, ...
    'x', zeros(1,MAX_len), 'y', zeros(1,MAX_len), 'yaw', zeros(1,MAX_len), ...
    'ds', zeros(1,MAX_len), 'kappa', zeros(1,MAX_len), ...
    'len', 0);

    fplist = repmat(fp_templet, 1, LENG_path);  % 빈 구조체 배열로 초기화
    index=1;
    for df = DF_SET
        for T = MIN_T:DT_T:MAX_T
            
            % Lateral trajectory (Quintic)
            [a0_d, a1_d, a2_d, a3_d, a4_d, a5_d] = calc_quintic(di, di_d, di_dd, df, df_d, df_dd, T);
            
            t = 0:DT:T;
            
            d = a0_d + a1_d*t + a2_d*t.^2 + a3_d*t.^3 + a4_d*t.^4 + a5_d*t.^5;
            d_d = a1_d + 2*a2_d*t + 3*a3_d*t.^2 + 4*a4_d*t.^3 + 5*a5_d*t.^4;
            d_dd = 2*a2_d + 6*a3_d*t + 12*a4_d*t.^2 + 20*a5_d*t.^3;
            d_ddd = 6*a3_d + 24*a4_d*t + 60*a5_d*t.^2;
            
            
            % Longitudinal trajectory (Quartic)
            %sf_d에 Target Speed를 기준으로 여러개 생성해야된다
            %sf 인자는 어디로 갔나
            [a0_s, a1_s, a2_s, a3_s, a4_s] = calc_quartic(si, si_d, si_dd, sf_d, sf_dd, T);
            s = a0_s + a1_s*t + a2_s*t.^2 + a3_s*t.^3 + a4_s*t.^4;
            s_d = a1_s + 2*a2_s*t + 3*a3_s*t.^2 + 4*a4_s*t.^3;
            s_dd = 2*a2_s + 6*a3_s*t + 12*a4_s*t.^2;
            s_ddd = 6*a3_s + 24*a4_s*t;
            
           
            %% 비용 계산
            J_lat = sum(d_ddd.^2); %적분항 인데 왜 T로 안나눠 임마 
            J_lon = sum(s_ddd.^2); %적분항 
            if gate_flag
                d_gate_weight = 10000000000;
                d_diff = (d(end) - TargetTolgateLane_d)^2 * d_gate_weight;
            else
                d_diff = (d(end) - opt_d)^2;
            end

            % if gate_flag
            %     opt_d = TargetTolgateLane_d;
            % else
            %     opt_d = di;
            % end


            s_diff = (TARGET_SPEED - s_d(end))^2; %ACC랑 최대한 유지하기 위함

            
            % if gate_flag
            %     d_gate_weight = 10000000000;
            %     d_diff = (d(end) - TargetTolgateLane_d)^2 * d_gate_weight;
            %     fprintf('[DEBUG] df = %.2f | d(end) = %.2f | target_d = %.2f | cost = %.2e\n', ...
            %             df, d(end), TargetTolgateLane_d, d_diff);
            % else
            %     d_diff = (d(end) - opt_d)^2;
            % end

            %% 비용함수
            c_lat = K_J * J_lat  + K_D * d_diff + K_T * T; %% cost_lateral
            c_lon = K_J * J_lon  + K_V * s_diff + K_T * T; %% cost_longitual
            c_tot = W_LAT * c_lat + W_LON * c_lon; %% total Cost가 낮은것을 선택

            len = length(t);  % ← 이 줄이 꼭 필요!

            % 1. fp 템플릿 기반 새 구조체 생성
            fp = fp_templet;

            % 2. 유효 길이 저장
            fp.len = len;

            % 3. 시간 및 궤적 데이터 복사
            fp.t(1:len)     = t;
            fp.d(1:len)     = d;
            fp.d_d(1:len)   = d_d;
            fp.d_dd(1:len)  = d_dd;
            fp.d_ddd(1:len) = d_ddd;

            fp.s(1:len)     = s;
            fp.s_d(1:len)   = s_d;
            fp.s_dd(1:len)  = s_dd;
            fp.s_ddd(1:len) = s_ddd;

            % 4. 비용도 할당
            fp.c_lat = c_lat;
            fp.c_lon = c_lon;
            fp.c_tot = c_tot;

            % 5. fplist에 대입
            fplist(index) = fp;
            if(index<LENG_path)
            index = index +1;
            end
        end
    end
end

function fplist = calc_global_paths(fplist, mapx, mapy, s_ref)
    for i = 1:length(fplist)
        fp = fplist(i);
        len = fp.len;

        % === Global 좌표 변환 === %
        for j = 1:len
            [fp.x(j), fp.y(j), ~] = get_cartesian(fp.s(j), fp.d(j), mapx, mapy, s_ref);
        end

        % === Yaw, ds 계산 === %
        for j = 1:len-1
            dx = fp.x(j+1) - fp.x(j);
            dy = fp.y(j+1) - fp.y(j);
            fp.yaw(j) = atan2(dy, dx);
            fp.ds(j) = hypot(dx, dy);
        end
        if len >= 2
            fp.yaw(len) = fp.yaw(len - 1);
            fp.ds(len)  = fp.ds(len - 1);
        else
            fp.yaw(len) = 0;
            fp.ds(len)  = 1e-6;  % 너무 작지 않게 보호
        end

        % === 곡률 계산 === %
        for j = 1:len-1
            dyaw = atan2(sin(fp.yaw(j+1) - fp.yaw(j)), cos(fp.yaw(j+1) - fp.yaw(j)));
            fp.kappa(j) = dyaw / fp.ds(j);
        end
        if len >= 2
            fp.kappa(len) = fp.kappa(len - 1);
        else
            fp.kappa(len) = 0;
        end

        % 업데이트된 fp 구조체 다시 저장
        fplist(i) = fp;
    end
end

function [valid_paths, numValid] = check_path(fplist, obs, MAX_len, LENG_path)
    % 정적 템플릿 구조체 선언
    fp_templet = struct( ...
        't', zeros(1,MAX_len), ...
        'd', zeros(1,MAX_len), 'd_d', zeros(1,MAX_len), 'd_dd', zeros(1,MAX_len), 'd_ddd', zeros(1,MAX_len), ...
        's', zeros(1,MAX_len), 's_d', zeros(1,MAX_len), 's_dd', zeros(1,MAX_len), 's_ddd', zeros(1,MAX_len), ...
        'c_lat', 0, 'c_lon', 0, 'c_tot', 0, ...
        'x', zeros(1,MAX_len), 'y', zeros(1,MAX_len), 'yaw', zeros(1,MAX_len), ...
        'ds', zeros(1,MAX_len), 'kappa', zeros(1,MAX_len), ...
        'len', 0);

    % 제약 조건
    V_MAX = 30;
    ACC_MAX = 5;
    K_MAX = 1.5;

    % 고정 크기 구조체 배열 선언
    valid_paths = repmat(fp_templet, 1, LENG_path);
    index = 1;
    numValid = 0;

    for i = 1:length(fplist)
        fp = fplist(i);
        len = fp.len;

        acc_squared = fp.s_dd(1:len).^2;  % s 방향에 대한 가속도만 고려
        

        if all(fp.s_d(1:len) > V_MAX)

            continue;
        % elseif any(acc_squared > ACC_MAX^2)
        %     continue;
        elseif any(abs(fp.kappa(1:len)) > K_MAX)
            continue;
        elseif collision_check(fp, obs)
            continue;
        elseif any(abs(fp.d(1:len)) > 3.5)
            continue;
        else
            valid_paths(index) = fp;
            index = index + 1;
            numValid = numValid + 1;
        end
    end

end


function collision = collision_check(fp, obs_global)
    CAR_RADIUS = 2;
    OBSTACLE_RADIUS = 0.5;
    SAFE_DIST_SQ = (CAR_RADIUS + OBSTACLE_RADIUS)^2;

    len = fp.len;
    collision = false;

    for i = 1:size(obs_global, 1)
        dx = fp.x(1:len) - obs_global(i,1);
        dy = fp.y(1:len) - obs_global(i,2);
        dists_sq = dx.^2 + dy.^2;

        if any(dists_sq <= SAFE_DIST_SQ)
            collision = true;
            return;
        end
    end
end



function [s, d] = get_frenet(x, y, x_ref, y_ref)
    idx = get_closest_waypoint(x, y, x_ref, y_ref);
    if idx == 1
        prev_idx = 1; next_idx = 2;
    elseif idx == length(x_ref)
        prev_idx = length(x_ref) - 1; next_idx = length(x_ref);
    else
        prev_idx = idx - 1; next_idx = idx;
    end
    vec_path = [x_ref(next_idx) - x_ref(prev_idx); y_ref(next_idx) - y_ref(prev_idx)];
    vec_ego  = [x - x_ref(prev_idx); y - y_ref(prev_idx)];
    proj = dot(vec_path, vec_ego) / norm(vec_path)^2 * vec_path;
    perp = vec_ego - proj;
    d = norm(perp);
    if det([vec_path, vec_ego]) < 0
        d = -d;
    end
    s = 0;
    for i = 1:(prev_idx - 1)
        s = s + norm([x_ref(i+1) - x_ref(i), y_ref(i+1) - y_ref(i)]);
    end
    s = s + norm(proj);
end

function [x, y, heading] = get_cartesian(s, d, x_ref, y_ref, s_ref)
    s = mod(s, s_ref(end));
    idx = find(s_ref <= s, 1, 'last');
    if idx >= length(s_ref), idx = length(s_ref) - 1; end
    dx = x_ref(idx+1) - x_ref(idx);
    dy = y_ref(idx+1) - y_ref(idx);
    heading = atan2(dy, dx);
    ds = s - s_ref(idx);
    x_base = x_ref(idx) + ds * cos(heading);
    y_base = y_ref(idx) + ds * sin(heading);
    x = x_base + d * cos(heading + pi/2);
    y = y_base + d * sin(heading + pi/2);
end

function idx = get_closest_waypoint(x, y, x_ref, y_ref)
    dists = sqrt((x_ref - x).^2 + (y_ref - y).^2);
    [~, idx] = min(dists);
end

function [a0, a1, a2, a3, a4, a5] = calc_quintic(xi, vi, ai, xf, vf, af, T)
    a0 = xi;
    a1 = vi;
    a2 = 0.5 * ai;
    A = [T^3, T^4, T^5;
         3*T^2, 4*T^3, 5*T^4;
         6*T, 12*T^2, 20*T^3];
    b = [xf - a0 - a1*T - a2*T^2;
         vf - a1 - 2*a2*T;
         af - 2*a2];
    x = A\b;
    a3 = x(1); a4 = x(2); a5 = x(3);
end

function [a0, a1, a2, a3, a4] = calc_quartic(xi, vi, ai, vf, af, T)
    a0 = xi;
    a1 = vi;
    a2 = 0.5 * ai;
    A = [3*T^2, 4*T^3;
         6*T, 12*T^2];
    b = [vf - a1 - 2*a2*T;
         af - 2*a2];
    x = A\b;
    a3 = x(1); a4 = x(2);
end

== matlab function generic_IVS/CarMaker/Subsystem/Final Project1/Scenario 1/Enabled Subsystem/MATLAB Function11 ==
  settings: updateMethod=DISCRETE  sampleTime=0.05
  data: traffic_info input; ego_pos input; ego_yaw input; ego_vx input; ego_lane_idx input; target_speed output; traffic_lane_idx input; debug_time_gap output; gate_flag input
function [target_speed, debug_time_gap] = acc_timegap_based( traffic_info,...
    ego_pos, ego_yaw, ego_vx, ego_lane_idx, ...
     traffic_lane_idx, gate_flag)

    % 기본 설정
    default_speed = 15.0;      % m/s (기본 크루즈 속도)
    safe_gap_time = 2.5;       % 안전 시간 간격 (초)
    emergency_gap_time = 1.8;  % 비상 시간 간격 (초)

    % 이전 속도 유지용 변수
    persistent last_speed
    if isempty(last_speed)
        last_speed = default_speed;
    end

    % 전방 차량 정보 분리
    traffic_pos = traffic_info(:, 1:2);   % 위치 [8x2]
    traffic_vx = traffic_info(:, 3);      % 속도 [8x1]
    L = size(traffic_info, 1);            % 차량 수

    % 초기값 설정
    min_gap_time = inf;
    front_vx = 0;
    found = false;

    ego_dir = [cos(ego_yaw); sin(ego_yaw)];  % 주행 방향 단위 벡터

    for i = 1:L
        if traffic_lane_idx(i) == ego_lane_idx
            dx = traffic_pos(i,1) - ego_pos(1);
            dy = traffic_pos(i,2) - ego_pos(2);
            rel_vec = [dx; dy];

            if dot(rel_vec, ego_dir) > 0  % 전방 차량인지 확인
                dist = norm(rel_vec);

                % ego 속도가 0이면 분모 0 방지
                if ego_vx > 0
                    time_gap = dist / ego_vx;
                else
                    time_gap = inf;
                end

                if time_gap < min_gap_time
                    min_gap_time = time_gap;
                    front_vx = traffic_vx(i);
                    found = true;
                end
            end
        end
    end

    % 기본 속도 계산 (gate_flag 고려 없이)
    speed = default_speed;
    if found
        if min_gap_time < emergency_gap_time
            speed = 0;  % 매우 위험 → 정지
        elseif min_gap_time < safe_gap_time
            ratio = (min_gap_time - emergency_gap_time) / (safe_gap_time - emergency_gap_time);
            speed = front_vx * ratio;
        end
    end

    % gate_flag에 따라 속도 조정
    if gate_flag
        last_speed = speed * 0.5;  % 속도 절반으로 줄이기
    else
        last_speed = speed;        % 원래 속도 복구
    end

    target_speed = last_speed;

    % 디버깅 정보 출력용
    debug_time_gap = min_gap_time;
end


% function [target_speed, debug_time_gap] = acc_timegap_based( ...
%     ego_pos, ego_yaw, ego_vx, ego_lane_idx, ...
%     traffic_info, traffic_lane_idx, gate_flag)
% 
% 
%     % 기본 설정
%     default_speed = 15.0;      % m/s (기본 크루즈 속도)
%     safe_gap_time = 2.5;       % 안전 시간 간격 (초)
%     emergency_gap_time = 1.8;  % 비상 시간 간격 (초)
% 
%     % 전방 차량 정보 분리
%     traffic_pos = traffic_info(:, 1:2);   % 위치 [8x2]
%     traffic_vx = traffic_info(:, 3);      % 속도 [8x1]
%     L = size(traffic_info, 1);            % 차량 수
% 
%     % 초기값 설정
%     min_gap_time = inf;
%     front_vx = 0;
%     found = false;
% 
%     ego_dir = [cos(ego_yaw); sin(ego_yaw)];  % 주행 방향 단위 벡터
% 
%     for i = 1:L
%         if traffic_lane_idx(i) == ego_lane_idx
%             dx = traffic_pos(i,1) - ego_pos(1);
%             dy = traffic_pos(i,2) - ego_pos(2);
%             rel_vec = [dx; dy];
% 
%             if dot(rel_vec, ego_dir) > 0  % 전방 차량인지 확인
%                 dist = norm(rel_vec);
% 
%                 % ego 속도가 0이면 분모 0 방지
%                 if ego_vx > 0
%                     time_gap = dist / ego_vx;
%                 else
%                     time_gap = inf;
%                 end
% 
%                 if time_gap < min_gap_time
%                     min_gap_time = time_gap;
%                     front_vx = traffic_vx(i);
%                     found = true;
%                 end
%             end
%         end
%     end
% 
%     % 속도 결정 로직
%     target_speed = default_speed;
% 
%     if found
%         if min_gap_time < emergency_gap_time
%             target_speed = 0;  % 매우 위험 → 정지
%         elseif min_gap_time < safe_gap_time
%             ratio = (min_gap_time - emergency_gap_time) / (safe_gap_time - emergency_gap_time);
%             target_speed = front_vx * ratio;
%         else
%             target_speed = default_speed;
%         end
%     end
% 
%     if gate_flag ==1
% 
%     % 디버깅 정보 출력용
%     debug_time_gap = min_gap_time;
% end
% 
%
